simulink model "Week_9_10_2r_robot_Simulation_Control - Copy"  (R2023a)
settings: Solver=ode4  StartTime=0.0  StopTime=20  FixedStep=1e-3  RelTol=1e-3  EnableMultiTasking=on
values from neighbouring files (symbols this model uses):
  g = zeros(1,2)    [puma560.m]    (also in willowRobotIK.m)
undefined symbols (not defined in the file or in its folder): l1, l2, m1, m2
libraries: dspinverses x3, slpidlib x2, dspfdesign x2
settings Model: Creator=e27269  LastModifiedBy=s3818101
settings SolverCC: AlgebraicLoopSolver=TrustRegion
settings DataIOCC: LimitDataPoints=on  ReturnWorkspaceOutputs=off
settings OptimizationCC: LifeSpan=inf
settings DebuggingCC: UnconnectedInputMsg=warning  UnconnectedOutputMsg=warning  UnconnectedLineMsg=warning  AllowSymbolicDim=off  SFUnexpectedBacktrackingDiag=warning  SFNoUnconditionalDefaultTransitionDiag=warning  SFExecutionAtInitializationDiag=none  ArithmeticOperatorsInVariantConditions=warning
settings ModelReferenceCC: EnableRefExpFcnMdlSchedulingChecks=on  PropagateSignalLabelsOutOfModel=off
settings SFSimCC: SimUseLocalCustomCode=off  CustomCodeUndefinedFunction=UseInterfaceOnly
settings RTWCC: RTWUseLocalCustomCode=off
settings CodeAppCC: StateflowObjectComments=on
settings GRTTargetCC: TargetLangStandard=C89/C90 (ANSI)
settings ConfigComp: CovMetricSettings=dw  CovSaveCumulativeToWorkspaceVar=on  CovSaveSingleToWorkspaceVar=on  CovExternalEMLEnable=off

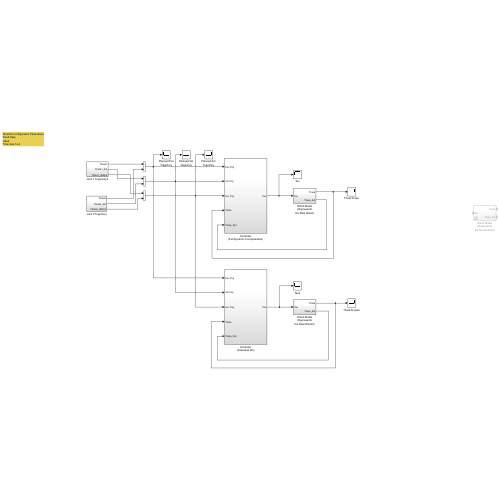
[thumbnail: Simulink's stored preview of the top-level diagram]
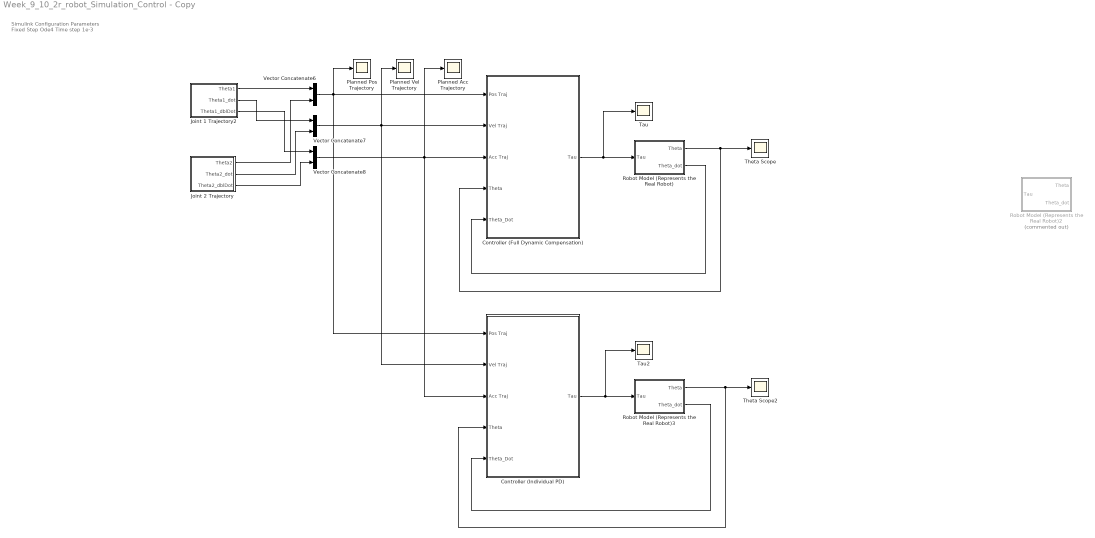
== system Week_9_10_2r_robot_Simulation_Control - Copy ==
  note: Simulink Configuration Parameters
      | Fixed Step
      | Ode4
      | Time step 1e-3
  Controller (Full Dynamic Compensation) : Subsystem
  Controller (Individual PD) : Subsystem
  Joint 1 Trajectory2 : Subsystem
  Joint 2 Trajectory : Subsystem
  Planned Acc Trajectory : Scope
  Planned Pos Trajectory : Scope
  Planned Vel Trajectory : Scope
  Robot Model (Represents the Real Robot) : Subsystem
  Robot Model (Represents the Real Robot)2 : Subsystem  Commented=on
  Robot Model (Represents the Real Robot)3 : Subsystem
  Tau : Scope
  Tau2 : Scope
  Theta Scope : Scope
  Theta Scope2 : Scope
  Vector Concatenate6 : Concatenate  Mode=Multidimensional array
  Vector Concatenate7 : Concatenate  Mode=Multidimensional array
  Vector Concatenate8 : Concatenate  Mode=Multidimensional array
  wires:
  Joint 1 Trajectory2/1(Theta1) -> Vector Concatenate6/1
  Joint 2 Trajectory/2(Theta2_dot) -> Vector Concatenate7/2
  Joint 2 Trajectory/1(Theta2) -> Vector Concatenate6/2
  Joint 1 Trajectory2/2(Theta1_dot) -> Vector Concatenate7/1
  Joint 1 Trajectory2/3(Theta1_dblDot) -> Vector Concatenate8/1
  Joint 2 Trajectory/3(Theta2_dblDot) -> Vector Concatenate8/2
  Vector Concatenate6/1 -> Controller (Individual PD)/1(Pos Traj), Controller (Full Dynamic Compensation)/1(Pos Traj), Planned Pos Trajectory/1
  Vector Concatenate7/1 -> Controller (Individual PD)/2(Vel Traj), Planned Vel Trajectory/1, Controller (Full Dynamic Compensation)/2(Vel Traj)
  Robot Model (Represents the Real Robot)/1(Theta) -> Controller (Full Dynamic Compensation)/4(Theta), Theta Scope/1
  Vector Concatenate8/1 -> Controller (Individual PD)/3(Acc Traj), Planned Acc Trajectory/1, Controller (Full Dynamic Compensation)/3(Acc Traj)
  Controller (Full Dynamic Compensation)/1(Tau) -> Tau/1, Robot Model (Represents the Real Robot)/1(Tau)
  Robot Model (Represents the Real Robot)/2(Theta_dot) -> Controller (Full Dynamic Compensation)/5(Theta_Dot)
  Robot Model (Represents the Real Robot)3/2(Theta_dot) -> Controller (Individual PD)/5(Theta_Dot)
  Controller (Individual PD)/1(Tau) -> Robot Model (Represents the Real Robot)3/1(Tau), Tau2/1
  Robot Model (Represents the Real Robot)3/1(Theta) -> Controller (Individual PD)/4(Theta), Theta Scope2/1

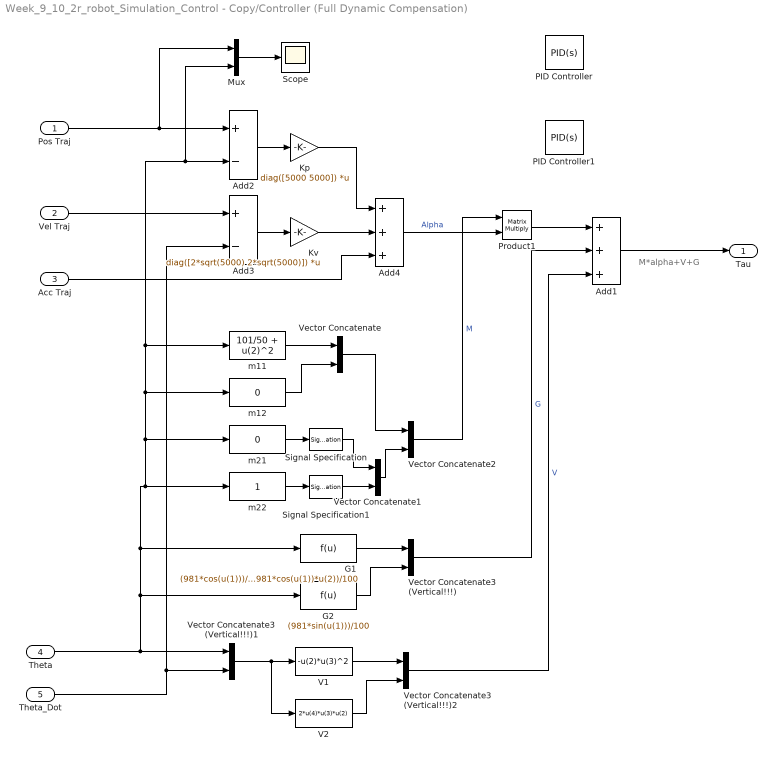
== system Week_9_10_2r_robot_Simulation_Control - Copy/Controller (Full Dynamic Compensation) ==
  note: M*alpha+V+G
  Pos Traj : Inport
  Vel Traj : Inport  Port=2
  Acc Traj : Inport  Port=3
  Theta : Inport  Port=4
  Theta_Dot : Inport  Port=5
  Add1 : Sum  Inputs=+++
  Add2 : Sum  Inputs=+-
  Add3 : Sum  Inputs=+-
  Add4 : Sum  Inputs=+++
  G1 : Fcn  Expr=(981*cos(u(1)))/500 + (981*cos(u(1))*u(2))/100
  G2 : Fcn  Expr=(981*sin(u(1)))/100
  Kp : Gain  Gain=diag([5000 5000])  Multiplication=Matrix(K*u) (u vector)
  Kv : Gain  Gain=diag([2*sqrt(5000) 2*sqrt(5000)])  Multiplication=Matrix(K*u) (u vector)
  Mux : Mux  Inputs=2
  PID Controller : slpidlib/PID Controller  Controller=PID  Form=Parallel  TimeDomain=Continuous-time  UseExternalTs=off  SampleTime=-1  IntegratorMethod=Forward Euler  FilterMethod=Forward Euler  ControllerParametersSource=internal  P=300  I=0  UseKiTs=off  D=0  N=100  UseFilter=on  TunerSelectOption=Transfer Function Based (PID Tuner App)  InitialConditionSource=internal  InitialConditionForIntegrator=0  InitialConditionForFilter=0  DifferentiatorICPrevScaledInput=0  ExternalReset=none  TrackingMode=off  Kt=1  LimitOutput=off  SatLimitsSource=internal  UpperSaturationLimit=inf  LowerSaturationLimit=-inf  LinearizeAsGain=on  AntiWindupMode=none  Kb=1  LimitIntegrator=off  UpperIntegratorSaturationLimit=inf  LowerIntegratorSaturationLimit=-inf  POutMin=[]  POutMax=[]  IOutMin=[]  IOutMax=[]  DOutMin=[]  DOutMax=[]  NOutMin=[]  NOutMax=[]  SumOutMin=[]  SumOutMax=[]  SaturationOutMin=[]  SaturationOutMax=[]  PParamMin=[]  PParamMax=[]  IParamMin=[]  IParamMax=[]  DParamMin=[]  DParamMax=[]  NParamMin=[]  NParamMax=[]  KbParamMin=[]  KbParamMax=[]  KtParamMin=[]  KtParamMax=[]  KbOutMin=[]  KbOutMax=[]  KtOutMin=[]  KtOutMax=[]  IntegratorOutMin=[]  IntegratorOutMax=[]  FilterOutMin=[]  FilterOutMax=[]  SumI1OutMin=[]  SumI1OutMax=[]  SumI2OutMin=[]  SumI2OutMax=[]  SumI3OutMin=[]  SumI3OutMax=[]  SumI4OutMin=[]  SumI4OutMax=[]  SumDOutMin=[]  SumDOutMax=[]  DifferentiatorOutMin=[]  DifferentiatorOutMax=[]  FilterDiffOutCoefMin=[]  FilterDiffOutCoefMax=[]  ReciprocalOutMin=[]  ReciprocalOutMax=[]  SumDenOutMin=[]  SumDenOutMax=[]  SumNumOutMin=[]  SumNumOutMax=[]  DivideOutMin=[]  DivideOutMax=[]  UdiffTsProdOutMin=[]  UdiffTsProdOutMax=[]  NTsProdOutMin=[]  NTsProdOutMax=[]  UintegralTsProdOutMin=[]  UintegralTsProdOutMax=[]  UngainTsProdOutMin=[]  UngainTsProdOutMax=[]  ClampingZeroOutDataTypeStr=Inherit: Inherit via back propagation  ClampingZeroOutMin=[]  ClampingZeroOutMax=[]  FilterDenConstantOutDataTypeStr=Inherit: Inherit via back propagation  FilterDenConstantOutMin=[]  FilterDenConstantOutMax=[]  PCopyOutDataTypeStr=Inherit: Inherit via back propagation  PCopyOutMin=[]  PCopyOutMax=[]  NCopyOutDataTypeStr=Inherit: Inherit via back propagation  NCopyOutMin=[]  NCopyOutMax=[]  IntegratorContinuousStateAttributes=''  IntegratorStateMustResolveToSignalObject=off  IntegratorRTWStateStorageClass=Auto  FilterContinuousStateAttributes=''  FilterStateMustResolveToSignalObject=off  FilterRTWStateStorageClass=Auto  ParallelPVariant=InternalParameters  IdealPVariant=Disabled  IVariant=InternalParameters  DVariant=InternalParameters  IntegratorVariant=Continuous  SatVariant=Disabled  AWVariant=Passthrough  PCopyVariant=Disabled  TRVariant=Disabled  FdbkBlocksVariant=Forward  IdealPFdbkVariant=Disabled  SatFdbkVariant=Disabled  DerivativeFilterVariant=ContFilter  NVariant=InternalParameters  NCopyVariant=Disabled  FilterICVariant=InternalICsFilter  IntegratorICVariant=InternalICs  ExternalResetVariant=Disabled  TRSumVariant=Passthrough  SumFdbkVariant=Disabled  SumVariant=Sum_PID  TsampFilterVariant=InternalTs  TsampNgainVariant=Passthrough  TsampIntegralVariant=Disabled_SignalSpec  ExternalSaturationOutDataTypeStr=Inherit: Same as second input
  PID Controller1 : slpidlib/PID Controller  Controller=PID  Form=Parallel  TimeDomain=Continuous-time  UseExternalTs=off  SampleTime=-1  IntegratorMethod=Forward Euler  FilterMethod=Forward Euler  ControllerParametersSource=internal  P=10  I=0  UseKiTs=off  D=0  N=100  UseFilter=on  TunerSelectOption=Transfer Function Based (PID Tuner App)  InitialConditionSource=internal  InitialConditionForIntegrator=0  InitialConditionForFilter=0  DifferentiatorICPrevScaledInput=0  ExternalReset=none  TrackingMode=off  Kt=1  LimitOutput=off  SatLimitsSource=internal  UpperSaturationLimit=inf  LowerSaturationLimit=-inf  LinearizeAsGain=on  AntiWindupMode=none  Kb=1  LimitIntegrator=off  UpperIntegratorSaturationLimit=inf  LowerIntegratorSaturationLimit=-inf  POutMin=[]  POutMax=[]  IOutMin=[]  IOutMax=[]  DOutMin=[]  DOutMax=[]  NOutMin=[]  NOutMax=[]  SumOutMin=[]  SumOutMax=[]  SaturationOutMin=[]  SaturationOutMax=[]  PParamMin=[]  PParamMax=[]  IParamMin=[]  IParamMax=[]  DParamMin=[]  DParamMax=[]  NParamMin=[]  NParamMax=[]  KbParamMin=[]  KbParamMax=[]  KtParamMin=[]  KtParamMax=[]  KbOutMin=[]  KbOutMax=[]  KtOutMin=[]  KtOutMax=[]  IntegratorOutMin=[]  IntegratorOutMax=[]  FilterOutMin=[]  FilterOutMax=[]  SumI1OutMin=[]  SumI1OutMax=[]  SumI2OutMin=[]  SumI2OutMax=[]  SumI3OutMin=[]  SumI3OutMax=[]  SumI4OutMin=[]  SumI4OutMax=[]  SumDOutMin=[]  SumDOutMax=[]  DifferentiatorOutMin=[]  DifferentiatorOutMax=[]  FilterDiffOutCoefMin=[]  FilterDiffOutCoefMax=[]  ReciprocalOutMin=[]  ReciprocalOutMax=[]  SumDenOutMin=[]  SumDenOutMax=[]  SumNumOutMin=[]  SumNumOutMax=[]  DivideOutMin=[]  DivideOutMax=[]  UdiffTsProdOutMin=[]  UdiffTsProdOutMax=[]  NTsProdOutMin=[]  NTsProdOutMax=[]  UintegralTsProdOutMin=[]  UintegralTsProdOutMax=[]  UngainTsProdOutMin=[]  UngainTsProdOutMax=[]  ClampingZeroOutDataTypeStr=Inherit: Inherit via back propagation  ClampingZeroOutMin=[]  ClampingZeroOutMax=[]  FilterDenConstantOutDataTypeStr=Inherit: Inherit via back propagation  FilterDenConstantOutMin=[]  FilterDenConstantOutMax=[]  PCopyOutDataTypeStr=Inherit: Inherit via back propagation  PCopyOutMin=[]  PCopyOutMax=[]  NCopyOutDataTypeStr=Inherit: Inherit via back propagation  NCopyOutMin=[]  NCopyOutMax=[]  IntegratorContinuousStateAttributes=''  IntegratorStateMustResolveToSignalObject=off  IntegratorRTWStateStorageClass=Auto  FilterContinuousStateAttributes=''  FilterStateMustResolveToSignalObject=off  FilterRTWStateStorageClass=Auto  ParallelPVariant=InternalParameters  IdealPVariant=Disabled  IVariant=InternalParameters  DVariant=InternalParameters  IntegratorVariant=Continuous  SatVariant=Disabled  AWVariant=Passthrough  PCopyVariant=Disabled  TRVariant=Disabled  FdbkBlocksVariant=Forward  IdealPFdbkVariant=Disabled  SatFdbkVariant=Disabled  DerivativeFilterVariant=ContFilter  NVariant=InternalParameters  NCopyVariant=Disabled  FilterICVariant=InternalICsFilter  IntegratorICVariant=InternalICs  ExternalResetVariant=Disabled  TRSumVariant=Passthrough  SumFdbkVariant=Disabled  SumVariant=Sum_PID  TsampFilterVariant=InternalTs  TsampNgainVariant=Passthrough  TsampIntegralVariant=Disabled_SignalSpec  ExternalSaturationOutDataTypeStr=Inherit: Same as second input
  Product1 : Product  Multiplication=Matrix(*)
  Scope : Scope
  Signal Specification : SignalSpecification  Dimensions=[1,1]
  Signal Specification1 : SignalSpecification  Dimensions=[1,1]
  V1 : Fcn  Expr=-u(2)*u(3)^2
  V2 : Fcn  Expr=2*u(4)*u(3)*u(2)
  Vector Concatenate : Concatenate  Mode=Multidimensional array  ConcatenateDimension=2
  Vector Concatenate1 : Concatenate  Mode=Multidimensional array  ConcatenateDimension=2
  Vector Concatenate2 : Concatenate  Mode=Multidimensional array
  Vector Concatenate3 (Vertical!!!) : Concatenate  Mode=Multidimensional array
  Vector Concatenate3 (Vertical!!!)1 : Concatenate  Mode=Multidimensional array
  Vector Concatenate3 (Vertical!!!)2 : Concatenate  Mode=Multidimensional array
  m11 : Fcn  Expr="101/50 +  u(2)^2"
  m12 : Fcn  Expr=0
  m21 : Fcn  Expr=0
  m22 : Fcn  Expr=1
  Tau : Outport  VectorParamsAs1DForOutWhenUnconnected=off
  wires:
  Vector Concatenate3 (Vertical!!!)2/1 -> Add1/3  "V"
  Vector Concatenate3 (Vertical!!!)1/1 -> V2/1, V1/1
  Theta_Dot/1 -> Vector Concatenate3 (Vertical!!!)1/2, Add3/2
  V1/1 -> Vector Concatenate3 (Vertical!!!)2/1
  Pos Traj/1 -> Mux/1, Add2/1
  Signal Specification/1 -> Vector Concatenate1/1
  Vel Traj/1 -> Add3/1
  V2/1 -> Vector Concatenate3 (Vertical!!!)2/2
  Vector Concatenate1/1 -> Vector Concatenate2/2
  Vector Concatenate/1 -> Vector Concatenate2/1
  Signal Specification1/1 -> Vector Concatenate1/2
  m12/1 -> Vector Concatenate/2
  G2/1 -> Vector Concatenate3 (Vertical!!!)/2
  G1/1 -> Vector Concatenate3 (Vertical!!!)/1
  Vector Concatenate2/1 -> Product1/1  "M"
  Acc Traj/1 -> Add4/3
  m22/1 -> Signal Specification1/1
  m11/1 -> Vector Concatenate/1
  m21/1 -> Signal Specification/1
  Add1/1 -> Tau/1
  Vector Concatenate3 (Vertical!!!)/1 -> Add1/2  "G"
  Product1/1 -> Add1/1
  Add2/1 -> Kp/1
  Add3/1 -> Kv/1
  Kv/1 -> Add4/2
  Kp/1 -> Add4/1
  Add4/1 -> Product1/2  "Alpha"
  Theta/1 -> Mux/2, Add2/2, m11/1, m12/1, m21/1, m22/1, G1/1, G2/1, Vector Concatenate3 (Vertical!!!)1/1
  Mux/1 -> Scope/1

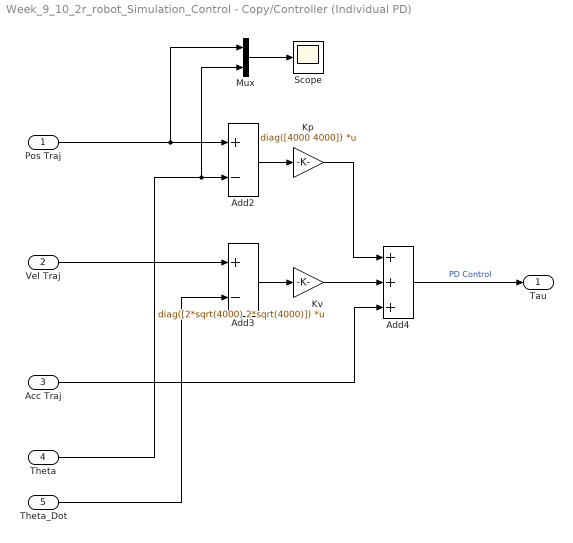
== system Week_9_10_2r_robot_Simulation_Control - Copy/Controller (Individual PD) ==
  Pos Traj : Inport
  Vel Traj : Inport  Port=2
  Acc Traj : Inport  Port=3
  Theta : Inport  Port=4
  Theta_Dot : Inport  Port=5
  Add2 : Sum  Inputs=+-
  Add3 : Sum  Inputs=+-
  Add4 : Sum  Inputs=+++
  Kp : Gain  Gain=diag([4000 4000])  Multiplication=Matrix(K*u) (u vector)
  Kv : Gain  Gain=diag([2*sqrt(4000) 2*sqrt(4000)])  Multiplication=Matrix(K*u) (u vector)
  Mux : Mux  Inputs=2
  Scope : Scope
  Tau : Outport  VectorParamsAs1DForOutWhenUnconnected=off
  wires:
  Theta_Dot/1 -> Add3/2
  Pos Traj/1 -> Mux/1, Add2/1
  Theta/1 -> Mux/2, Add2/2
  Vel Traj/1 -> Add3/1
  Acc Traj/1 -> Add4/3
  Add2/1 -> Kp/1
  Add3/1 -> Kv/1
  Kv/1 -> Add4/2
  Kp/1 -> Add4/1
  Add4/1 -> Tau/1  "PD Control"
  Mux/1 -> Scope/1

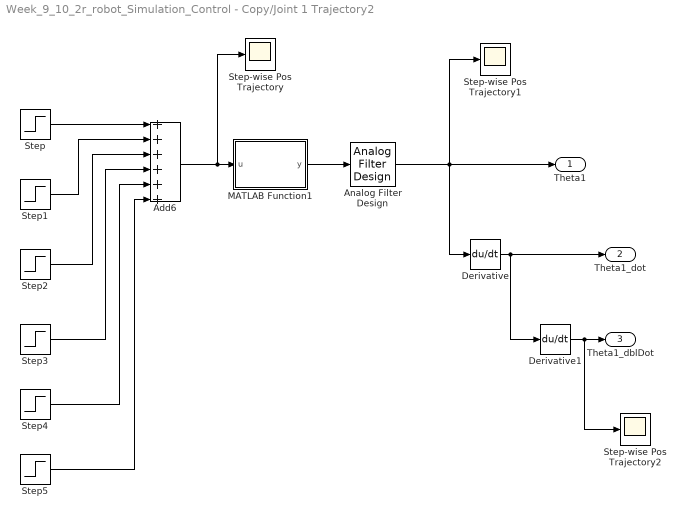
== system Week_9_10_2r_robot_Simulation_Control - Copy/Joint 1 Trajectory2 ==
  Add6 : Sum  Inputs=6
  Analog Filter Design : dspfdesign/Analog Filter Design  method=Butterworth  filttype=Lowpass  N=1  Wlo=20  Whi=80  Rp=2  Rs=40
  Derivative : Derivative
  Derivative1 : Derivative
  MATLAB Function1 : MATLAB Function  TreatAsAtomicUnit=on
  Step : Step  SampleTime=0
  Step-wise Pos Trajectory : Scope
  Step-wise Pos Trajectory1 : Scope
  Step-wise Pos Trajectory2 : Scope
  Step1 : Step  Time=4  After=2  SampleTime=0
  Step2 : Step  Time=8  After=-1  SampleTime=0
  Step3 : Step  Time=11  After=1.5  SampleTime=0
  Step4 : Step  Time=14  After=-1  SampleTime=0
  Step5 : Step  Time=17  After=-2  SampleTime=0
  Theta1 : Outport  VectorParamsAs1DForOutWhenUnconnected=off
  Theta1_dot : Outport  Port=2  VectorParamsAs1DForOutWhenUnconnected=off
  Theta1_dblDot : Outport  Port=3  VectorParamsAs1DForOutWhenUnconnected=off
  wires:
  Step/1 -> Add6/1
  Add6/1 -> MATLAB Function1/1(u), Step-wise Pos Trajectory/1
  Step5/1 -> Add6/6
  Step3/1 -> Add6/4
  Step4/1 -> Add6/5
  Step1/1 -> Add6/2
  Step2/1 -> Add6/3
  Derivative/1 -> Derivative1/1, Theta1_dot/1
  Derivative1/1 -> Step-wise Pos Trajectory2/1, Theta1_dblDot/1
  MATLAB Function1/1(y) -> Analog Filter Design/1
  Analog Filter Design/1 -> Step-wise Pos Trajectory1/1, Derivative/1, Theta1/1

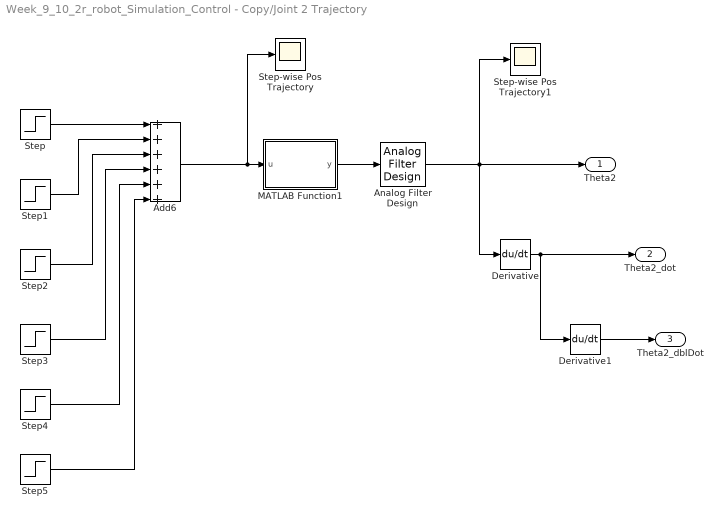
== system Week_9_10_2r_robot_Simulation_Control - Copy/Joint 2 Trajectory ==
  Add6 : Sum  Inputs=6
  Analog Filter Design : dspfdesign/Analog Filter Design  method=Butterworth  filttype=Lowpass  N=1  Wlo=20  Whi=80  Rp=2  Rs=40
  Derivative : Derivative
  Derivative1 : Derivative
  MATLAB Function1 : MATLAB Function  TreatAsAtomicUnit=on
  Step : Step  After=0.5  SampleTime=0
  Step-wise Pos Trajectory : Scope
  Step-wise Pos Trajectory1 : Scope
  Step1 : Step  Time=4  After=1.5  SampleTime=0
  Step2 : Step  Time=8  After=-1  SampleTime=0
  Step3 : Step  Time=12  After=2.5  SampleTime=0
  Step4 : Step  Time=16  After=0.5  SampleTime=0
  Step5 : Step  Time=18  After=-2  SampleTime=0
  Theta2 : Outport  VectorParamsAs1DForOutWhenUnconnected=off
  Theta2_dot : Outport  Port=2  VectorParamsAs1DForOutWhenUnconnected=off
  Theta2_dblDot : Outport  Port=3  VectorParamsAs1DForOutWhenUnconnected=off
  wires:
  Step2/1 -> Add6/3
  Step1/1 -> Add6/2
  Step4/1 -> Add6/5
  Step3/1 -> Add6/4
  Step5/1 -> Add6/6
  Step/1 -> Add6/1
  Derivative/1 -> Theta2_dot/1, Derivative1/1
  Analog Filter Design/1 -> Theta2/1, Step-wise Pos Trajectory1/1, Derivative/1
  Add6/1 -> MATLAB Function1/1(u), Step-wise Pos Trajectory/1
  MATLAB Function1/1(y) -> Analog Filter Design/1
  Derivative1/1 -> Theta2_dblDot/1

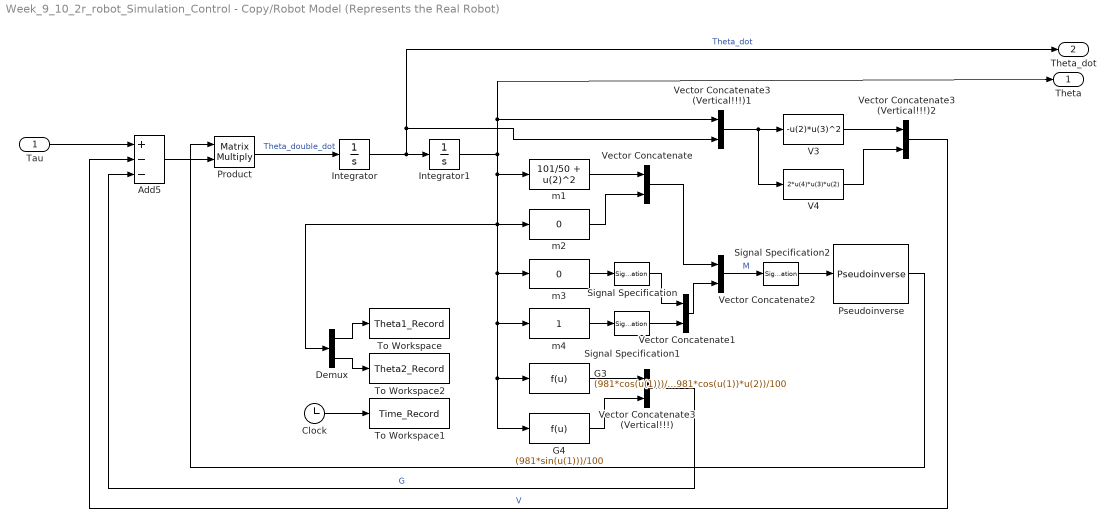
== system Week_9_10_2r_robot_Simulation_Control - Copy/Robot Model (Represents the Real Robot) ==
  Tau : Inport
  Add5 : Sum  Inputs=+--
  Clock : Clock
  Demux : Demux  Outputs=2
  G3 : Fcn  Expr=(981*cos(u(1)))/500 + (981*cos(u(1))*u(2))/100
  G4 : Fcn  Expr=(981*sin(u(1)))/100
  Integrator : Integrator  InitialCondition=[0;0]
  Integrator1 : Integrator  InitialCondition=[0;0.5]
  Product : Product  Multiplication=Matrix(*)
  Pseudoinverse : dspinverses/Pseudoinverse  wanterr=off  SimulateUsing=Interpreted execution
  Signal Specification : SignalSpecification  Dimensions=[1,1]
  Signal Specification1 : SignalSpecification  Dimensions=[1,1]
  Signal Specification2 : SignalSpecification  Dimensions=[2,2]
  To Workspace : ToWorkspace  VariableName=Theta1_Record  SampleTime=-1
      settings: Save2DSignal=2-D array (concatenate along first dimension)
  To Workspace1 : ToWorkspace  VariableName=Time_Record  SampleTime=-1
      settings: Save2DSignal=2-D array (concatenate along first dimension)
  To Workspace2 : ToWorkspace  VariableName=Theta2_Record  SampleTime=-1
      settings: Save2DSignal=2-D array (concatenate along first dimension)
  V3 : Fcn  Expr=-u(2)*u(3)^2
  V4 : Fcn  Expr=2*u(4)*u(3)*u(2)
  Vector Concatenate : Concatenate  Mode=Multidimensional array  ConcatenateDimension=2
  Vector Concatenate1 : Concatenate  Mode=Multidimensional array  ConcatenateDimension=2
  Vector Concatenate2 : Concatenate  Mode=Multidimensional array
  Vector Concatenate3 (Vertical!!!) : Concatenate  Mode=Multidimensional array
  Vector Concatenate3 (Vertical!!!)1 : Concatenate  Mode=Multidimensional array
  Vector Concatenate3 (Vertical!!!)2 : Concatenate  Mode=Multidimensional array
  m1 : Fcn  Expr="101/50 +  u(2)^2"
  m2 : Fcn  Expr=0
  m3 : Fcn  Expr=0
  m4 : Fcn  Expr=1
  Theta : Outport  VectorParamsAs1DForOutWhenUnconnected=off
  Theta_dot : Outport  Port=2  VectorParamsAs1DForOutWhenUnconnected=off
  wires:
  Tau/1 -> Add5/1
  Integrator/1 -> Theta_dot/1, Vector Concatenate3 (Vertical!!!)1/2, Integrator1/1  "Theta_dot"
  Product/1 -> Integrator/1  "Theta_double_dot"
  Integrator1/1 -> m1/1, m2/1, Demux/1, m3/1, m4/1, G3/1, G4/1, Theta/1, Vector Concatenate3 (Vertical!!!)1/1
  m1/1 -> Vector Concatenate/1
  m2/1 -> Vector Concatenate/2
  m3/1 -> Signal Specification/1
  m4/1 -> Signal Specification1/1
  Vector Concatenate1/1 -> Vector Concatenate2/2
  Vector Concatenate/1 -> Vector Concatenate2/1
  Vector Concatenate2/1 -> Signal Specification2/1  "M"
  G3/1 -> Vector Concatenate3 (Vertical!!!)/1
  G4/1 -> Vector Concatenate3 (Vertical!!!)/2
  Vector Concatenate3 (Vertical!!!)/1 -> Add5/3  "G"
  V3/1 -> Vector Concatenate3 (Vertical!!!)2/1
  V4/1 -> Vector Concatenate3 (Vertical!!!)2/2
  Vector Concatenate3 (Vertical!!!)2/1 -> Add5/2  "V"
  Add5/1 -> Product/2
  Pseudoinverse/1 -> Product/1
  Signal Specification/1 -> Vector Concatenate1/1
  Signal Specification1/1 -> Vector Concatenate1/2
  Signal Specification2/1 -> Pseudoinverse/1
  Clock/1 -> To Workspace1/1
  Demux/1 -> To Workspace/1
  Demux/2 -> To Workspace2/1
  Vector Concatenate3 (Vertical!!!)1/1 -> V4/1, V3/1

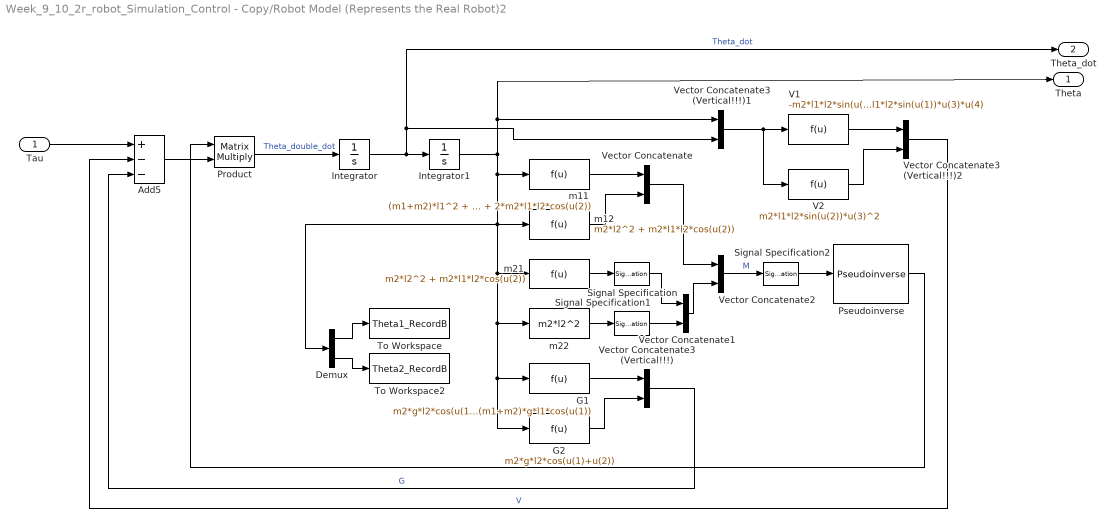
== system Week_9_10_2r_robot_Simulation_Control - Copy/Robot Model (Represents the Real Robot)2 ==
  Tau : Inport
  Add5 : Sum  Inputs=+--
  Demux : Demux  Outputs=2
  G1 : Fcn  Expr=m2*g*l2*cos(u(1)+u(2))+(m1+m2)*g*l1*cos(u(1))
  G2 : Fcn  Expr=m2*g*l2*cos(u(1)+u(2))
  Integrator : Integrator  InitialCondition=[0;0]
  Integrator1 : Integrator  InitialCondition=[0;0.5]
  Product : Product  Multiplication=Matrix(*)
  Pseudoinverse : dspinverses/Pseudoinverse  wanterr=off  SimulateUsing=Interpreted execution
  Signal Specification : SignalSpecification  Dimensions=[1,1]
  Signal Specification1 : SignalSpecification  Dimensions=[1,1]
  Signal Specification2 : SignalSpecification  Dimensions=[2,2]
  To Workspace : ToWorkspace  VariableName=Theta1_RecordB  SampleTime=-1
      settings: Save2DSignal=2-D array (concatenate along first dimension)
  To Workspace2 : ToWorkspace  VariableName=Theta2_RecordB  SampleTime=-1
      settings: Save2DSignal=2-D array (concatenate along first dimension)
  V1 : Fcn  Expr=-m2*l1*l2*sin(u(2))*u(4)^2-2*m2*l1*l2*sin(u(1))*u(3)*u(4)
  V2 : Fcn  Expr=m2*l1*l2*sin(u(2))*u(3)^2
  Vector Concatenate : Concatenate  Mode=Multidimensional array  ConcatenateDimension=2
  Vector Concatenate1 : Concatenate  Mode=Multidimensional array  ConcatenateDimension=2
  Vector Concatenate2 : Concatenate  Mode=Multidimensional array
  Vector Concatenate3 (Vertical!!!) : Concatenate  Mode=Multidimensional array
  Vector Concatenate3 (Vertical!!!)1 : Concatenate  Mode=Multidimensional array
  Vector Concatenate3 (Vertical!!!)2 : Concatenate  Mode=Multidimensional array
  m11 : Fcn  Expr=(m1+m2)*l1^2 + m2*l2^2 + 2*m2*l1*l2*cos(u(2))
  m12 : Fcn  Expr=m2*l2^2 + m2*l1*l2*cos(u(2))
  m21 : Fcn  Expr=m2*l2^2 + m2*l1*l2*cos(u(2))
  m22 : Fcn  Expr=m2*l2^2
  Theta : Outport  VectorParamsAs1DForOutWhenUnconnected=off
  Theta_dot : Outport  Port=2  VectorParamsAs1DForOutWhenUnconnected=off
  wires:
  Tau/1 -> Add5/1
  Integrator/1 -> Theta_dot/1, Vector Concatenate3 (Vertical!!!)1/2, Integrator1/1  "Theta_dot"
  Product/1 -> Integrator/1  "Theta_double_dot"
  Integrator1/1 -> Demux/1, m12/1, m21/1, m22/1, G1/1, G2/1, m11/1, Theta/1, Vector Concatenate3 (Vertical!!!)1/1
  m11/1 -> Vector Concatenate/1
  m12/1 -> Vector Concatenate/2
  m21/1 -> Signal Specification/1
  m22/1 -> Signal Specification1/1
  Vector Concatenate1/1 -> Vector Concatenate2/2
  Vector Concatenate/1 -> Vector Concatenate2/1
  Vector Concatenate2/1 -> Signal Specification2/1  "M"
  G1/1 -> Vector Concatenate3 (Vertical!!!)/1
  G2/1 -> Vector Concatenate3 (Vertical!!!)/2
  Vector Concatenate3 (Vertical!!!)/1 -> Add5/3  "G"
  Vector Concatenate3 (Vertical!!!)1/1 -> V2/1, V1/1
  V1/1 -> Vector Concatenate3 (Vertical!!!)2/1
  V2/1 -> Vector Concatenate3 (Vertical!!!)2/2
  Vector Concatenate3 (Vertical!!!)2/1 -> Add5/2  "V"
  Add5/1 -> Product/2
  Pseudoinverse/1 -> Product/1
  Signal Specification/1 -> Vector Concatenate1/1
  Signal Specification1/1 -> Vector Concatenate1/2
  Signal Specification2/1 -> Pseudoinverse/1
  Demux/1 -> To Workspace/1
  Demux/2 -> To Workspace2/1

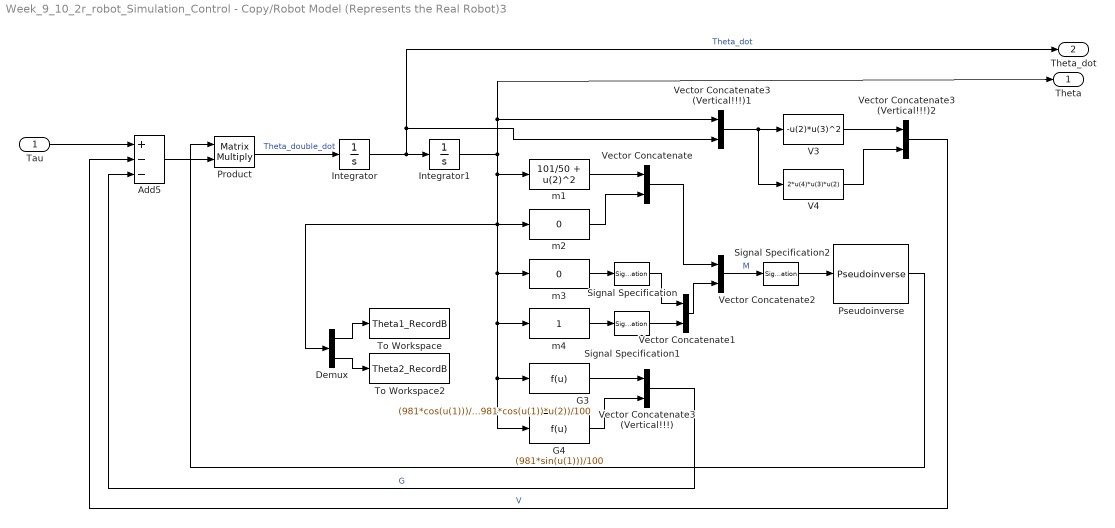
== system Week_9_10_2r_robot_Simulation_Control - Copy/Robot Model (Represents the Real Robot)3 ==
  Tau : Inport
  Add5 : Sum  Inputs=+--
  Demux : Demux  Outputs=2
  G3 : Fcn  Expr=(981*cos(u(1)))/500 + (981*cos(u(1))*u(2))/100
  G4 : Fcn  Expr=(981*sin(u(1)))/100
  Integrator : Integrator  InitialCondition=[0;0]
  Integrator1 : Integrator  InitialCondition=[0;0.5]
  Product : Product  Multiplication=Matrix(*)
  Pseudoinverse : dspinverses/Pseudoinverse  wanterr=off  SimulateUsing=Interpreted execution
  Signal Specification : SignalSpecification  Dimensions=[1,1]
  Signal Specification1 : SignalSpecification  Dimensions=[1,1]
  Signal Specification2 : SignalSpecification  Dimensions=[2,2]
  To Workspace : ToWorkspace  VariableName=Theta1_RecordB  SampleTime=-1
      settings: Save2DSignal=2-D array (concatenate along first dimension)
  To Workspace2 : ToWorkspace  VariableName=Theta2_RecordB  SampleTime=-1
      settings: Save2DSignal=2-D array (concatenate along first dimension)
  V3 : Fcn  Expr=-u(2)*u(3)^2
  V4 : Fcn  Expr=2*u(4)*u(3)*u(2)
  Vector Concatenate : Concatenate  Mode=Multidimensional array  ConcatenateDimension=2
  Vector Concatenate1 : Concatenate  Mode=Multidimensional array  ConcatenateDimension=2
  Vector Concatenate2 : Concatenate  Mode=Multidimensional array
  Vector Concatenate3 (Vertical!!!) : Concatenate  Mode=Multidimensional array
  Vector Concatenate3 (Vertical!!!)1 : Concatenate  Mode=Multidimensional array
  Vector Concatenate3 (Vertical!!!)2 : Concatenate  Mode=Multidimensional array
  m1 : Fcn  Expr="101/50 +  u(2)^2"
  m2 : Fcn  Expr=0
  m3 : Fcn  Expr=0
  m4 : Fcn  Expr=1
  Theta : Outport  VectorParamsAs1DForOutWhenUnconnected=off
  Theta_dot : Outport  Port=2  VectorParamsAs1DForOutWhenUnconnected=off
  wires:
  Tau/1 -> Add5/1
  Integrator/1 -> Theta_dot/1, Vector Concatenate3 (Vertical!!!)1/2, Integrator1/1  "Theta_dot"
  Product/1 -> Integrator/1  "Theta_double_dot"
  Integrator1/1 -> m1/1, m2/1, Demux/1, m3/1, m4/1, G3/1, G4/1, Theta/1, Vector Concatenate3 (Vertical!!!)1/1
  m1/1 -> Vector Concatenate/1
  m2/1 -> Vector Concatenate/2
  m3/1 -> Signal Specification/1
  m4/1 -> Signal Specification1/1
  Vector Concatenate1/1 -> Vector Concatenate2/2
  Vector Concatenate/1 -> Vector Concatenate2/1
  Vector Concatenate2/1 -> Signal Specification2/1  "M"
  G3/1 -> Vector Concatenate3 (Vertical!!!)/1
  G4/1 -> Vector Concatenate3 (Vertical!!!)/2
  Vector Concatenate3 (Vertical!!!)/1 -> Add5/3  "G"
  V3/1 -> Vector Concatenate3 (Vertical!!!)2/1
  V4/1 -> Vector Concatenate3 (Vertical!!!)2/2
  Vector Concatenate3 (Vertical!!!)2/1 -> Add5/2  "V"
  Add5/1 -> Product/2
  Pseudoinverse/1 -> Product/1
  Signal Specification/1 -> Vector Concatenate1/1
  Signal Specification1/1 -> Vector Concatenate1/2
  Signal Specification2/1 -> Pseudoinverse/1
  Demux/1 -> To Workspace/1
  Demux/2 -> To Workspace2/1
  Vector Concatenate3 (Vertical!!!)1/1 -> V4/1, V3/1

== matlab function Week_9_10_2r_robot_Simulation_Control - Copy/Joint 2 Trajectory/MATLAB Function1 ==
  settings: updateMethod=DISCRETE
  data: u input; y output
function y = average_filter(u)
 order =1000;
persistent filter_buffer 
if isempty(filter_buffer)   
    filter_buffer = zeros(1,order);
end

for i=order:-1:2
    filter_buffer(1,i) = filter_buffer(1,i-1);
end

filter_buffer(1,1) = u;

% output of the average filter
y = sum(filter_buffer)/order;
% y= filter_buffer;

== matlab function Week_9_10_2r_robot_Simulation_Control - Copy/Joint 1 Trajectory2/MATLAB Function1 ==
  settings: updateMethod=DISCRETE
  data: u input; y output
function y = average_filter(u)
 order =1000;
persistent filter_buffer 
if isempty(filter_buffer)   
    filter_buffer = zeros(1,order);
end

for i=order:-1:2
    filter_buffer(1,i) = filter_buffer(1,i-1);
end

filter_buffer(1,1) = u;

% output of the average filter
y = sum(filter_buffer)/order;
% y= filter_buffer;
